simulink model "Simple_4Quad_payload_03"  (R2018b)
settings: Solver=VariableStepAuto  StartTime=0.0  StopTime=60  RelTol=1e-3
InitFcn:
  | Simple_4Quad_payload_03_const
values from neighbouring files (symbols this model uses):
  B = 1e0*eye(n)    [Simple_2Quad_payload_03_const.m]    (also in constant_CAMFC2_Quad_New_02_Payload_01.m = eye(n); test01.m = [eye(3) eye(3) eye(3) eye(3))
  BBT_inv = ((B'*B)^(-1))*B'    [Simple_2Quad_payload_03_const.m]    (also in Simple_4Quad_payload_04_const.m = ((BR'*BR)^(-1))*BR'; Simple_4Quad_payload_05_const.m = ((BR'*BR)^(-1))*BR'; Simple_4Quad_payload_06_const.m = ((BR'*BR)^(-1))*BR'; Simple_4Quad_payload_07_const.m = ((BR'*BR)^(-1))*BR')
  d1 = 0.25    [Colab_4Quad_model_01_const.m]    (also in Colab_4Quad_model_02_const.m = 0.5; Simple_4Quad_payload_01_const.m = 1; Simple_4Quad_payload_02_const.m = 1; Simple_4Quad_payload_03_const.m = 1)
  d2 = 0.25    [Colab_4Quad_model_01_const.m]    (also in Colab_4Quad_model_02_const.m = 0.5; Simple_4Quad_payload_01_const.m = 1; Simple_4Quad_payload_02_const.m = 1; Simple_4Quad_payload_03_const.m = 1)
  Des_rel_dist = 2    [Simple_4Quad_payload_01_const.m]    (also in Simple_4Quad_payload_02_const.m = 4; Simple_4Quad_payload_03_const.m = 4; Simple_4Quad_payload_04_const.m; Simple_4Quad_payload_05_const.m)
  gamma_0 = 1e-0*diag([1e-3;1e-0])    [Simple_2Quad_payload_03_const.m]    (also in Simple_4Quad_payload_04_const.m = 1e-0*diag([1e-6*ones(3,1);1e-0*ones(3,1)]); Simple_4Quad_payload_05_const.m = 1e-1*diag([1e-6*ones(3,1);1e-0*ones(3,1)]); Simple_4Quad_payload_06_const.m = 1e-0*diag([1e-6*ones(3,1);1e-0*ones(3,1)]); Simple_4Quad_payload_07_const.m = 1e-0*diag([1e-6*ones(3,1);1e-0*ones(3,1)]))
  gamma_1 = 1e+2*diag([1e-3;1e-0])    [Simple_2Quad_payload_03_const.m]    (also in Simple_4Quad_payload_04_const.m = 1e+2*diag([1e-6*ones(3,1);1e-0*ones(3,1)]); Simple_4Quad_payload_05_const.m = 1e+2*diag([1e-6*ones(3,1);1e-0*ones(3,1)]); Simple_4Quad_payload_06_const.m = 1e+3*diag([1e-6*ones(3,1);1e-0*ones(3,1)]); Simple_4Quad_payload_07_const.m = 1e+3*diag([1e-6*ones(3,1);1e-0*ones(3,1)]))
  ge = 9.81    [Simple_4Quad_payload_03_const.m]    (also in constant_CAMFC2_Quad_New_02_Payload_01.m)
  Ix = 0.166667    [Colab_4Quad_model_01_const.m]    (also in Colab_4Quad_model_02_const.m = 0.02; Simple_4Quad_payload_01_const.m = 1; Simple_4Quad_payload_02_const.m = 1; Simple_4Quad_payload_03_const.m = 1)
  Iy = 0.166667    [Colab_4Quad_model_01_const.m]    (also in Colab_4Quad_model_02_const.m = 0.02; Simple_4Quad_payload_01_const.m = 1; Simple_4Quad_payload_02_const.m = 1; Simple_4Quad_payload_03_const.m = 1)
  Iz = 0.166667    [Colab_4Quad_model_01_const.m]    (also in Colab_4Quad_model_02_const.m = 0.02; Simple_4Quad_payload_01_const.m = 1; Simple_4Quad_payload_02_const.m = 1; Simple_4Quad_payload_03_const.m = 1)
  Jq = diag([0.0291 0.0291 0.0552])    [Colab_4Quad_model_01_const.m]    (also in Colab_4Quad_model_02_const.m = diag([0.03 0.03 0.06]); Simple_4Quad_payload_03_const.m = 1.2416e-3 * diag([1 1 2]); Simple_4Quad_payload_04_const.m = 1 * diag([1 1 2]); Simple_4Quad_payload_05_const.m = 1 * diag([1 1 2]))
  k1 = 1    [Simple_2Quad_payload_03_const.m]    (also in Simple_4Quad_payload_04_const.m; Simple_4Quad_payload_05_const.m; Simple_4Quad_payload_06_const.m; Simple_4Quad_payload_07_const.m)
  k2 = 0.1    [Simple_2Quad_payload_03_const.m]    (also in Simple_4Quad_payload_04_const.m; Simple_4Quad_payload_05_const.m; Simple_4Quad_payload_06_const.m; Simple_4Quad_payload_07_const.m)
  Ka = 0.01    [Simple_4Quad_payload_03_const.m]    (also in constant_CAMFC2_Quad_New_02_Payload_01.m)
  Kd = 0.01    [Simple_4Quad_payload_03_const.m]    (also in constant_CAMFC2_Quad_New_02_Payload_01.m)
  Kf = 1.0e-5    (= 1e-05)    [Simple_4Quad_payload_03_const.m]    (also in constant_CAMFC2_Quad_New_02_Payload_01.m)
  ki1_N = 0    [Simple_4Quad_payload_02_const.m]    (also in Simple_4Quad_payload_03_const.m; Simple_4Quad_payload_04_const.m; Simple_4Quad_payload_05_const.m; Simple_4Quad_payload_06_const.m)
  ki1_S = 0    [Simple_4Quad_payload_02_const.m]    (also in Simple_4Quad_payload_03_const.m; Simple_4Quad_payload_04_const.m)
  ki2_N = 0    [Simple_4Quad_payload_02_const.m]    (also in Simple_4Quad_payload_03_const.m; Simple_4Quad_payload_04_const.m; Simple_4Quad_payload_05_const.m; Simple_4Quad_payload_06_const.m = 10)
  ki2_S = 0    [Simple_4Quad_payload_02_const.m]    (also in Simple_4Quad_payload_03_const.m; Simple_4Quad_payload_04_const.m)
  kp1_N = 10    [Simple_4Quad_payload_02_const.m]    (also in Simple_4Quad_payload_03_const.m; Simple_4Quad_payload_04_const.m; Simple_4Quad_payload_05_const.m = 1; Simple_4Quad_payload_06_const.m = 1)
  kp1_S = 10    [Simple_4Quad_payload_02_const.m]    (also in Simple_4Quad_payload_03_const.m; Simple_4Quad_payload_04_const.m)
  kp2_N = 100    [Simple_4Quad_payload_02_const.m]    (also in Simple_4Quad_payload_03_const.m; Simple_4Quad_payload_04_const.m; Simple_4Quad_payload_05_const.m = 1; Simple_4Quad_payload_06_const.m = 1)
  kp2_S = 100    [Simple_4Quad_payload_02_const.m]    (also in Simple_4Quad_payload_03_const.m; Simple_4Quad_payload_04_const.m)
  Kt = 0.0435 * Kf    (= 4.35e-07)    [Simple_4Quad_payload_03_const.m]    (also in constant_CAMFC2_Quad_New_02_Payload_01.m = 1e-07)
  l = 3.1819    [Colab_4Quad_model_01_const.m]    (also in Colab_4Quad_model_02_const.m = 3; Simple_2Quad_payload_04_const.m = 1; Simple_4Quad_payload_01_const.m = 1; Simple_4Quad_payload_02_const.m = 2)
  Lq = 0.45    [Simple_4Quad_payload_03_const.m]    (also in constant_CAMFC2_Quad_New_02_Payload_01.m = 0.2)
  m = 1.5    [Colab_4Quad_model_01_const.m]    (also in Colab_4Quad_model_02_const.m; Simple_2Quad_payload_04_const.m = 1; Simple_4Quad_payload_01_const.m = 1; Simple_4Quad_payload_02_const.m = 1)
  M = 1.0    (= 1)    [Colab_4Quad_model_01_const.m]    (also in Colab_4Quad_model_02_const.m; Simple_2Quad_payload_01_const.m; Simple_2Quad_payload_02_const.m; Simple_2Quad_payload_03_const.m)
  Md = 1*[1;1;1]    [Simple_2Quad_payload_04_const.m]    (also in Simple_4Quad_payload_01_const.m = 1*[1;1;1;1;1;1]; Simple_4Quad_payload_02_const.m = 1*[1;1;1;1;1;1]; Simple_4Quad_payload_03_const.m = 1*[1;1;1;1;1;1]; Simple_4Quad_payload_04_const.m = 1*[1;1;1;1;1;1])
  Mq = 2.95    [Simple_4Quad_payload_03_const.m]
  n = 2    [Simple_2Quad_payload_03_const.m]    (also in Simple_4Quad_payload_03_const.m = 6; Simple_4Quad_payload_04_const.m = 6; Simple_4Quad_payload_05_const.m = 6; Simple_4Quad_payload_06_const.m = 6)
  QR = 1e-0*eye(n)    [Simple_4Quad_payload_04_const.m]    (also in Simple_4Quad_payload_05_const.m = 1e-1*eye(n); Simple_4Quad_payload_06_const.m; Simple_4Quad_payload_07_const.m; Simple_4Quad_payload_08_const.m)
  R = 1e+0*eye(n)    [Simple_2Quad_payload_03_const.m]    (also in Simple_4Quad_payload_04_const.m = 1e+0*eye(m); Simple_4Quad_payload_05_const.m = 1e+0*eye(m); Simple_4Quad_payload_06_const.m; Simple_4Quad_payload_07_const.m)
  rho_0 = 1e-0    (= 1)    [Simple_2Quad_payload_03_const.m]    (also in Simple_4Quad_payload_04_const.m; Simple_4Quad_payload_05_const.m = 0.1; Simple_4Quad_payload_06_const.m; Simple_4Quad_payload_07_const.m)
  rho_1 = 1e-0    (= 1)    [Simple_2Quad_payload_03_const.m]    (also in Simple_4Quad_payload_04_const.m; Simple_4Quad_payload_05_const.m; Simple_4Quad_payload_06_const.m; Simple_4Quad_payload_07_const.m)
undefined symbols (not defined in the file or in its folder): mq
libraries: simulink x16
(part 1 of 3)
settings Model: Creator=ali  LastModifiedBy=ali

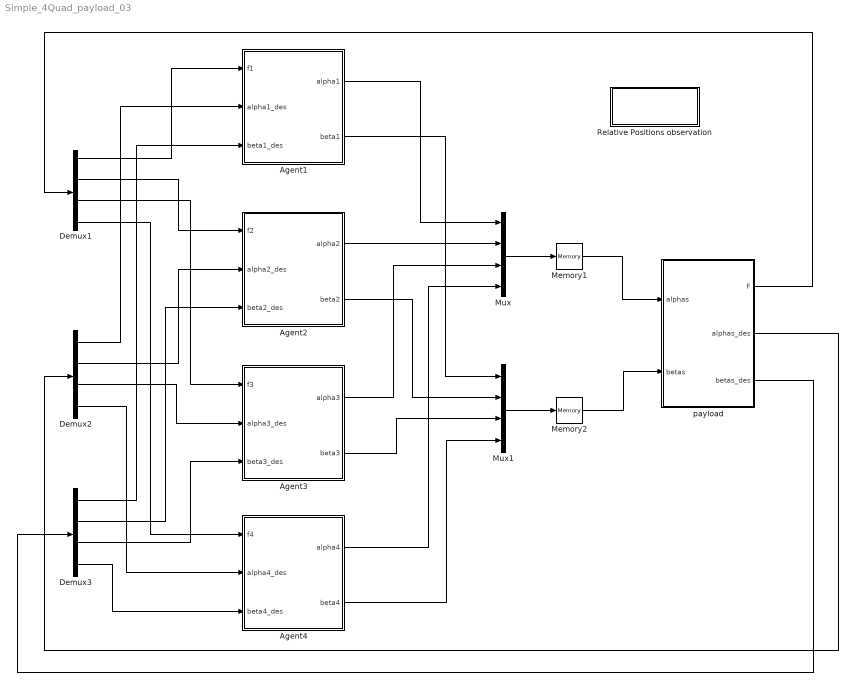
== system Simple_4Quad_payload_03 ==
  "Agent1 " : Subsystem
  Agent2 : Subsystem
  Agent3 : Subsystem
  Agent4 : Subsystem
  Demux1 : Demux
  Demux2 : Demux
  Demux3 : Demux
  Memory1 : Memory  InitialCondition=zeros(4,1)
  Memory2 : Memory  InitialCondition=zeros(4,1)
  Mux : Mux
  Mux1 : Mux
  Relative Positions observation : Subsystem
  payload : Subsystem
  wires:
  payload/1(F) -> Demux1/1
  payload/2(alphas_des) -> Demux2/1
  payload/3(betas_des) -> Demux3/1
  Demux1/1 -> "Agent1 "/1(f1)
  Demux1/2 -> Agent2/1(f2)
  Demux1/3 -> Agent3/1(f3)
  Demux1/4 -> Agent4/1(f4)
  Demux2/1 -> "Agent1 "/2(alpha1_des)
  Demux2/2 -> Agent2/2(alpha2_des)
  Demux2/3 -> Agent3/2(alpha3_des)
  Demux3/1 -> "Agent1 "/3(beta1_des)
  Demux3/2 -> Agent2/3(beta2_des)
  Demux3/3 -> Agent3/3(beta3_des)
  Demux2/4 -> Agent4/2(alpha4_des)
  Demux3/4 -> Agent4/3(beta4_des)
  "Agent1 "/1(alpha1) -> Mux/1
  Agent2/1(alpha2) -> Mux/2
  Agent3/1(alpha3) -> Mux/3
  Agent4/1(alpha4) -> Mux/4
  "Agent1 "/2(beta1) -> Mux1/1
  Agent2/2(beta2) -> Mux1/2
  Agent3/2(beta3) -> Mux1/3
  Agent4/2(beta4) -> Mux1/4
  Mux/1 -> Memory1/1
  Mux1/1 -> Memory2/1
  Memory2/1 -> payload/2(betas)
  Memory1/1 -> payload/1(alphas)

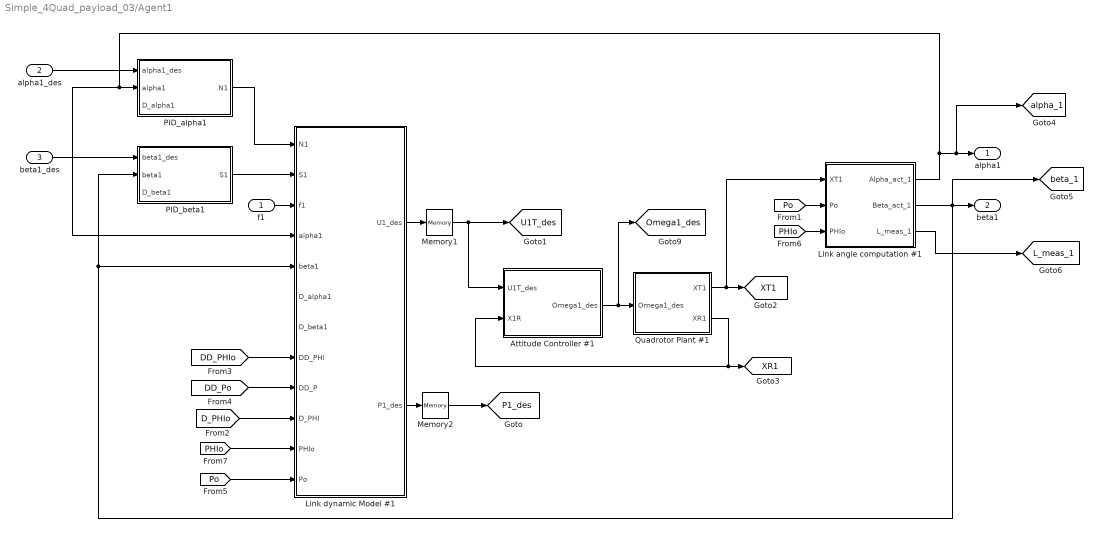
== system Simple_4Quad_payload_03/Agent1  ==
  f1 : Inport
  alpha1_des : Inport  Port=2
  beta1_des : Inport  Port=3
  Attitude Controller #1 : Subsystem
  Link angle computation #1 : MATLAB Function  TreatAsAtomicUnit=on
  Link dynamic Model #1 : MATLAB Function  TreatAsAtomicUnit=on
  Memory1 : Memory  InitialCondition=zeros(3,1)
  Memory2 : Memory  InitialCondition=zeros(3,1)
  PID_alpha1 : Subsystem
  PID_beta1 : Subsystem
  Quadrotor Plant #1 : Subsystem
  alpha1 : Outport
  beta1 : Outport  Port=2
  tag scope: L_meas_1=global, Omega1_des=global, P1_des=global, U1T_des=global, XR1=global, XT1=global, alpha_1=global, beta_1=global
  wires:
  PID_alpha1/1(N1) -> Link dynamic Model #1/1(N1)
  PID_beta1/1(S1) -> Link dynamic Model #1/2(S1)
  f1/1 -> Link dynamic Model #1/3(f1)
  Memory2/1 -> [P1_des]
  Memory1/1 -> Attitude Controller #1/1(U1T_des), [U1T_des]
  beta1_des/1 -> PID_beta1/1(beta1_des)
  [PHIo] -> Link dynamic Model #1/11(PHIo)
  [DD_Po] -> Link dynamic Model #1/9(DD_P)
  [D_PHIo] -> Link dynamic Model #1/10(D_PHI)
  [Po] -> Link dynamic Model #1/12(Po)
  [DD_PHIo] -> Link dynamic Model #1/8(DD_PHI)
  Link dynamic Model #1/1(U1_des) -> Memory1/1
  alpha1_des/1 -> PID_alpha1/1(alpha1_des)
  Link dynamic Model #1/2(P1_des) -> Memory2/1
  Quadrotor Plant #1/2(XR1) -> Attitude Controller #1/2(X1R), [XR1]
  Attitude Controller #1/1(Omega1_des) -> Quadrotor Plant #1/1(Omega1_des), [Omega1_des]
  Quadrotor Plant #1/1(XT1) -> Link angle computation #1/1(XT1), [XT1]
  Link angle computation #1/2(Beta_act_1) -> [beta_1], PID_beta1/2(beta1), Link dynamic Model #1/5(beta1), beta1/1
  Link angle computation #1/1(Alpha_act_1) -> Link dynamic Model #1/4(alpha1), PID_alpha1/2(alpha1), [alpha_1], alpha1/1
  [Po] -> Link angle computation #1/2(Po)
  [PHIo] -> Link angle computation #1/3(PHIo)
  Link angle computation #1/3(L_meas_1) -> [L_meas_1]

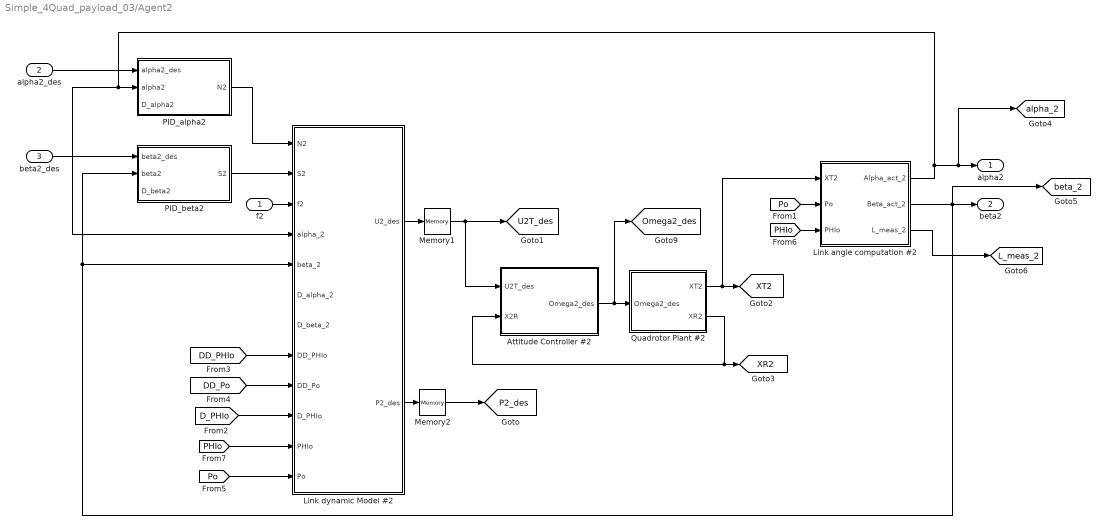
== system Simple_4Quad_payload_03/Agent2 ==
  f2 : Inport
  alpha2_des : Inport  Port=2
  beta2_des : Inport  Port=3
  Attitude Controller #2 : Subsystem
  Link angle computation #2 : MATLAB Function  TreatAsAtomicUnit=on
  Link dynamic Model #2 : MATLAB Function  TreatAsAtomicUnit=on
  Memory1 : Memory  InitialCondition=zeros(3,1)
  Memory2 : Memory  InitialCondition=zeros(3,1)
  PID_alpha2 : Subsystem
  PID_beta2 : Subsystem
  Quadrotor Plant #2 : Subsystem
  alpha2 : Outport
  beta2 : Outport  Port=2
  tag scope: L_meas_2=global, Omega2_des=global, P2_des=global, U2T_des=global, XR2=global, XT2=global, alpha_2=global, beta_2=global
  wires:
  PID_alpha2/1(N2) -> Link dynamic Model #2/1(N2)
  PID_beta2/1(S2) -> Link dynamic Model #2/2(S2)
  f2/1 -> Link dynamic Model #2/3(f2)
  Memory2/1 -> [P2_des]
  Memory1/1 -> Attitude Controller #2/1(U2T_des), [U2T_des]
  beta2_des/1 -> PID_beta2/1(beta2_des)
  [PHIo] -> Link dynamic Model #2/11(PHIo)
  [DD_Po] -> Link dynamic Model #2/9(DD_Po)
  [D_PHIo] -> Link dynamic Model #2/10(D_PHIo)
  [Po] -> Link dynamic Model #2/12(Po)
  [DD_PHIo] -> Link dynamic Model #2/8(DD_PHIo)
  Link dynamic Model #2/1(U2_des) -> Memory1/1
  alpha2_des/1 -> PID_alpha2/1(alpha2_des)
  Link dynamic Model #2/2(P2_des) -> Memory2/1
  Quadrotor Plant #2/2(XR2) -> Attitude Controller #2/2(X2R), [XR2]
  Attitude Controller #2/1(Omega2_des) -> Quadrotor Plant #2/1(Omega2_des), [Omega2_des]
  Quadrotor Plant #2/1(XT2) -> Link angle computation #2/1(XT2), [XT2]
  Link angle computation #2/2(Beta_act_2) -> [beta_2], PID_beta2/2(beta2), Link dynamic Model #2/5(beta_2), beta2/1
  Link angle computation #2/1(Alpha_act_2) -> Link dynamic Model #2/4(alpha_2), PID_alpha2/2(alpha2), [alpha_2], alpha2/1
  [Po] -> Link angle computation #2/2(Po)
  [PHIo] -> Link angle computation #2/3(PHIo)
  Link angle computation #2/3(L_meas_2) -> [L_meas_2]

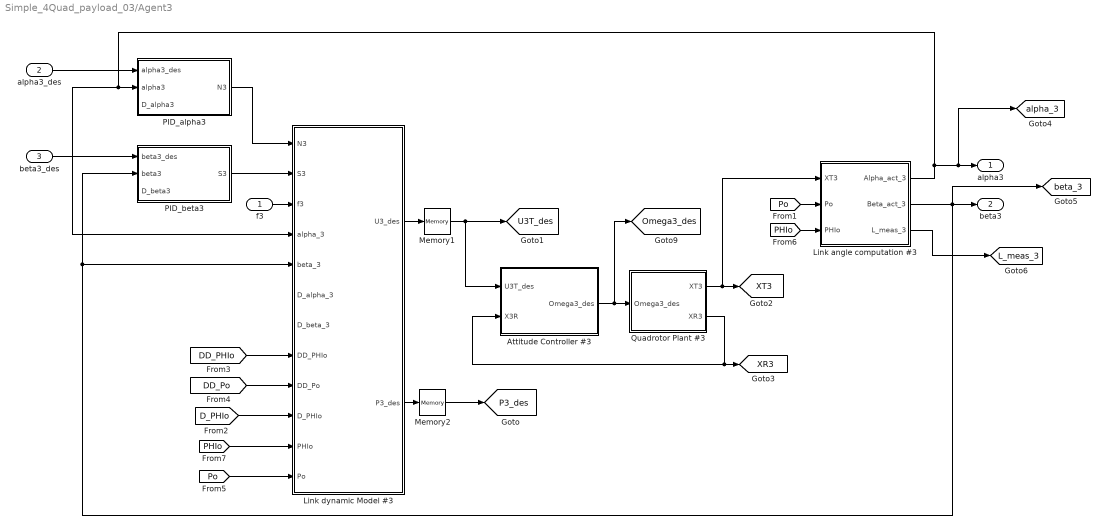
== system Simple_4Quad_payload_03/Agent3 ==
  f3 : Inport
  alpha3_des : Inport  Port=2
  beta3_des : Inport  Port=3
  Attitude Controller #3 : Subsystem
  Link angle computation #3 : MATLAB Function  TreatAsAtomicUnit=on
  Link dynamic Model #3 : MATLAB Function  TreatAsAtomicUnit=on
  Memory1 : Memory  InitialCondition=zeros(3,1)
  Memory2 : Memory  InitialCondition=zeros(3,1)
  PID_alpha3 : Subsystem
  PID_beta3 : Subsystem
  Quadrotor Plant #3 : Subsystem
  alpha3 : Outport
  beta3 : Outport  Port=2
  tag scope: L_meas_3=global, Omega3_des=global, P3_des=global, U3T_des=global, XR3=global, XT3=global, alpha_3=global, beta_3=global
  wires:
  Link angle computation #3/3(L_meas_3) -> [L_meas_3]
  [PHIo] -> Link angle computation #3/3(PHIo)
  [Po] -> Link angle computation #3/2(Po)
  Link angle computation #3/1(Alpha_act_3) -> alpha3/1, [alpha_3], PID_alpha3/2(alpha3), Link dynamic Model #3/4(alpha_3)
  Link angle computation #3/2(Beta_act_3) -> beta3/1, Link dynamic Model #3/5(beta_3), PID_beta3/2(beta3), [beta_3]
  Quadrotor Plant #3/1(XT3) -> [XT3], Link angle computation #3/1(XT3)
  Attitude Controller #3/1(Omega3_des) -> [Omega3_des], Quadrotor Plant #3/1(Omega3_des)
  Quadrotor Plant #3/2(XR3) -> [XR3], Attitude Controller #3/2(X3R)
  Link dynamic Model #3/2(P3_des) -> Memory2/1
  alpha3_des/1 -> PID_alpha3/1(alpha3_des)
  Link dynamic Model #3/1(U3_des) -> Memory1/1
  [DD_PHIo] -> Link dynamic Model #3/8(DD_PHIo)
  [Po] -> Link dynamic Model #3/12(Po)
  [D_PHIo] -> Link dynamic Model #3/10(D_PHIo)
  [DD_Po] -> Link dynamic Model #3/9(DD_Po)
  [PHIo] -> Link dynamic Model #3/11(PHIo)
  beta3_des/1 -> PID_beta3/1(beta3_des)
  Memory1/1 -> [U3T_des], Attitude Controller #3/1(U3T_des)
  Memory2/1 -> [P3_des]
  f3/1 -> Link dynamic Model #3/3(f3)
  PID_beta3/1(S3) -> Link dynamic Model #3/2(S3)
  PID_alpha3/1(N3) -> Link dynamic Model #3/1(N3)

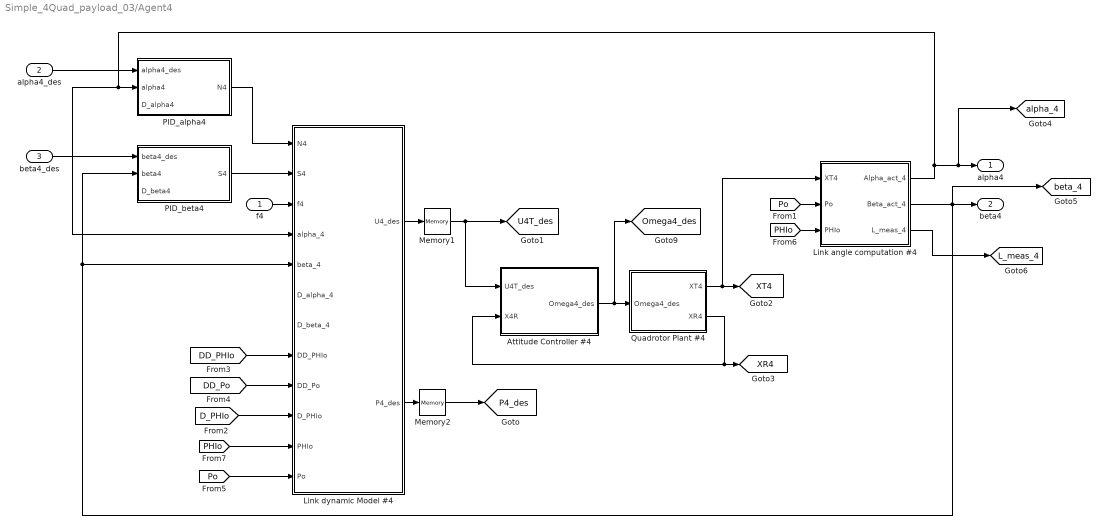
== system Simple_4Quad_payload_03/Agent4 ==
  f4 : Inport
  alpha4_des : Inport  Port=2
  beta4_des : Inport  Port=3
  Attitude Controller #4 : Subsystem
  Link angle computation #4 : MATLAB Function  TreatAsAtomicUnit=on
  Link dynamic Model #4 : MATLAB Function  TreatAsAtomicUnit=on
  Memory1 : Memory  InitialCondition=zeros(3,1)
  Memory2 : Memory  InitialCondition=zeros(3,1)
  PID_alpha4 : Subsystem
  PID_beta4 : Subsystem
  Quadrotor Plant #4 : Subsystem
  alpha4 : Outport
  beta4 : Outport  Port=2
  tag scope: L_meas_4=global, Omega4_des=global, P4_des=global, U4T_des=global, XR4=global, XT4=global, alpha_4=global, beta_4=global
  wires:
  PID_alpha4/1(N4) -> Link dynamic Model #4/1(N4)
  PID_beta4/1(S4) -> Link dynamic Model #4/2(S4)
  f4/1 -> Link dynamic Model #4/3(f4)
  Memory2/1 -> [P4_des]
  Memory1/1 -> Attitude Controller #4/1(U4T_des), [U4T_des]
  beta4_des/1 -> PID_beta4/1(beta4_des)
  [PHIo] -> Link dynamic Model #4/11(PHIo)
  [DD_Po] -> Link dynamic Model #4/9(DD_Po)
  [D_PHIo] -> Link dynamic Model #4/10(D_PHIo)
  [Po] -> Link dynamic Model #4/12(Po)
  [DD_PHIo] -> Link dynamic Model #4/8(DD_PHIo)
  Link dynamic Model #4/1(U4_des) -> Memory1/1
  alpha4_des/1 -> PID_alpha4/1(alpha4_des)
  Link dynamic Model #4/2(P4_des) -> Memory2/1
  Quadrotor Plant #4/2(XR4) -> Attitude Controller #4/2(X4R), [XR4]
  Attitude Controller #4/1(Omega4_des) -> Quadrotor Plant #4/1(Omega4_des), [Omega4_des]
  Quadrotor Plant #4/1(XT4) -> Link angle computation #4/1(XT4), [XT4]
  Link angle computation #4/2(Beta_act_4) -> [beta_4], PID_beta4/2(beta4), Link dynamic Model #4/5(beta_4), beta4/1
  Link angle computation #4/1(Alpha_act_4) -> Link dynamic Model #4/4(alpha_4), PID_alpha4/2(alpha4), [alpha_4], alpha4/1
  [Po] -> Link angle computation #4/2(Po)
  [PHIo] -> Link angle computation #4/3(PHIo)
  Link angle computation #4/3(L_meas_4) -> [L_meas_4]

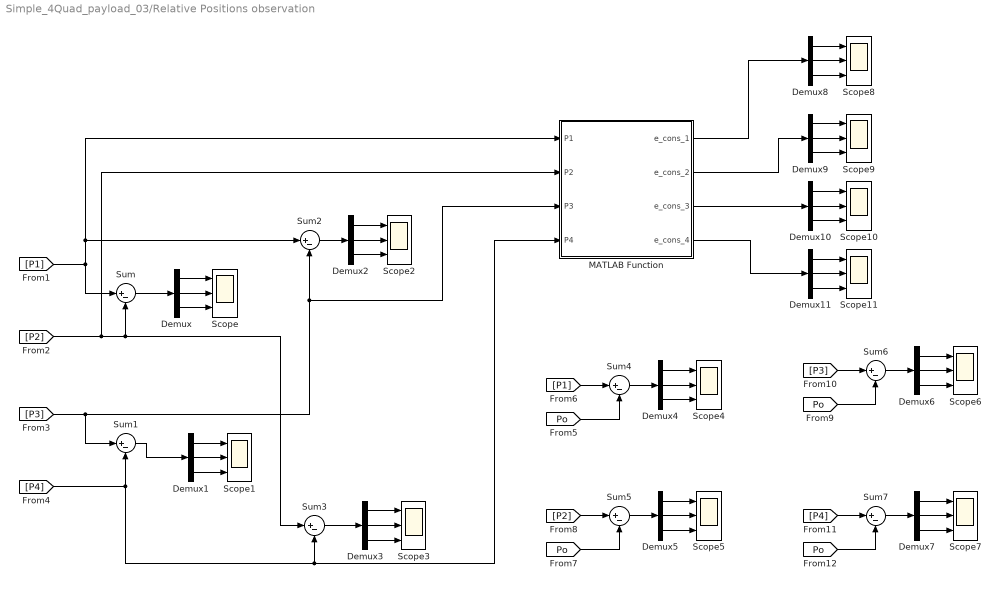
== system Simple_4Quad_payload_03/Relative Positions observation ==
  Demux{,1..11} (12 alike) : Demux  Outputs=3
  MATLAB Function : MATLAB Function  TreatAsAtomicUnit=on
  Scope{,1..11} (12 alike) : Scope  NumInputPorts=3
  Sum{,1..7} (8 alike) : Sum  Inputs=|+-
  wires:
  Demux/3 -> Scope/3
  Demux/1 -> Scope/1
  Demux/2 -> Scope/2
  Sum/1 -> Demux/1
  Sum1/1 -> Demux1/1
  Demux1/2 -> Scope1/2
  Demux1/1 -> Scope1/1
  Demux1/3 -> Scope1/3
  Sum2/1 -> Demux2/1
  [P3] -> MATLAB Function/3(P3), Sum2/2, Sum1/1
  [P1] -> Sum/1, MATLAB Function/1(P1), Sum2/1
  Demux2/2 -> Scope2/2
  Demux2/1 -> Scope2/1
  Demux2/3 -> Scope2/3
  Demux3/3 -> Scope3/3
  Demux3/1 -> Scope3/1
  Demux3/2 -> Scope3/2
  [P2] -> MATLAB Function/2(P2), Sum/2, Sum3/1
  [P4] -> Sum3/2, MATLAB Function/4(P4), Sum1/2
  Sum3/1 -> Demux3/1
  Demux4/3 -> Scope4/3
  Demux4/1 -> Scope4/1
  Demux4/2 -> Scope4/2
  Sum4/1 -> Demux4/1
  Sum5/1 -> Demux5/1
  Demux5/2 -> Scope5/2
  Demux5/1 -> Scope5/1
  Demux5/3 -> Scope5/3
  Demux6/3 -> Scope6/3
  Demux6/1 -> Scope6/1
  Demux6/2 -> Scope6/2
  Sum6/1 -> Demux6/1
  Sum7/1 -> Demux7/1
  Demux7/2 -> Scope7/2
  Demux7/1 -> Scope7/1
  Demux7/3 -> Scope7/3
  [Po] -> Sum4/2
  [P1] -> Sum4/1
  [P2] -> Sum5/1
  [Po] -> Sum5/2
  [P3] -> Sum6/1
  [Po] -> Sum6/2
  [P4] -> Sum7/1
  [Po] -> Sum7/2
  Demux8/2 -> Scope8/2
  Demux8/1 -> Scope8/1
  Demux8/3 -> Scope8/3
  MATLAB Function/1(e_cons_1) -> Demux8/1
  Demux9/3 -> Scope9/3
  Demux9/1 -> Scope9/1
  Demux9/2 -> Scope9/2
  MATLAB Function/2(e_cons_2) -> Demux9/1
  Demux10/2 -> Scope10/2
  Demux10/1 -> Scope10/1
  Demux10/3 -> Scope10/3
  MATLAB Function/3(e_cons_3) -> Demux10/1
  Demux11/3 -> Scope11/3
  Demux11/1 -> Scope11/1
  Demux11/2 -> Scope11/2
  MATLAB Function/4(e_cons_4) -> Demux11/1

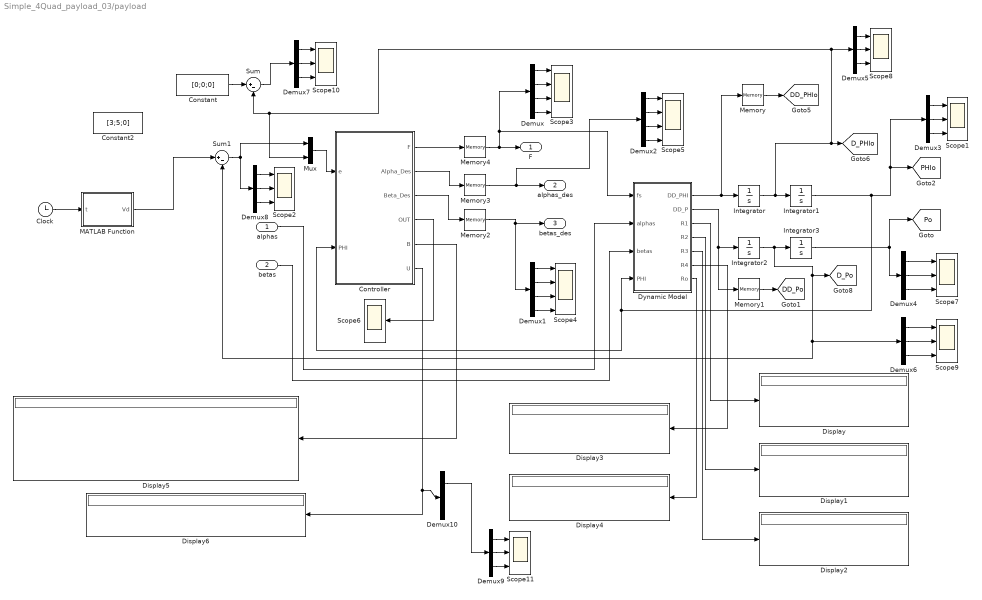
== system Simple_4Quad_payload_03/payload ==
  alphas : Inport
  betas : Inport  Port=2
  Clock : Clock
  Constant : Constant  Value=[0;0;0]
  Constant2 : Constant  Value=[3;5;0]
  Controller : MATLAB Function  TreatAsAtomicUnit=on
  Demux : Demux
  Demux1 : Demux
  Demux10 : Demux  Outputs=2
  Demux2 : Demux
  Demux{3..9} (7 alike) : Demux  Outputs=3
  Display{,1..6} (7 alike) : Display
  Dynamic Model : MATLAB Function  TreatAsAtomicUnit=on
  Integrator : Integrator  InitialCondition=zeros(3,1)
  Integrator1 : Integrator  InitialCondition=zeros(3,1)
  Integrator2 : Integrator  InitialCondition=zeros(3,1)
  Integrator3 : Integrator  InitialCondition=[0;0;0]
  MATLAB Function : MATLAB Function  TreatAsAtomicUnit=on
  Memory : Memory  InitialCondition=zeros(3,1)
  Memory1 : Memory  InitialCondition=zeros(3,1)
  Memory2 : Memory  InitialCondition=[0;pi;pi/2;-pi/2]
  Memory3 : Memory  InitialCondition=pi/2*ones(4,1)
  Memory4 : Memory  InitialCondition=zeros(4,1)
  Mux : Mux  Inputs=2
  Scope{1..2,7..11} (7 alike) : Scope  NumInputPorts=3
  Scope3 : Scope  NumInputPorts=4
  Scope4 : Scope  NumInputPorts=4
  Scope5 : Scope  NumInputPorts=4
  Scope6 : Scope
  Sum : Sum  Inputs=|+-
  Sum1 : Sum  Inputs=|+-
  F : Outport
  alphas_des : Outport  Port=2
  betas_des : Outport  Port=3
  tag scope: DD_PHIo=global, DD_Po=global, D_PHIo=global, D_Po=global, PHIo=global, Po=global
  wires:
  Dynamic Model/1(DD_PHI) -> Integrator/1, Memory/1
  Integrator/1 -> Integrator1/1, [D_PHIo], Demux5/1, Mux/2, Sum/2
  Integrator1/1 -> Demux3/1, [PHIo], Controller/2(PHI), Dynamic Model/4(PHI)
  Integrator2/1 -> Integrator3/1, [D_Po], Sum1/2, Demux6/1
  Dynamic Model/2(DD_P) -> Memory1/1, Integrator2/1
  alphas/1 -> Dynamic Model/2(alphas)
  Integrator3/1 -> [Po], Demux4/1
  Constant/1 -> Sum/1
  MATLAB Function/1(Vd) -> Sum1/1
  Memory/1 -> [DD_PHIo]
  Controller/4(OUT) -> Scope6/1
  Mux/1 -> Controller/1(e)
  betas/1 -> Dynamic Model/3(betas)
  Controller/1(F) -> Memory4/1
  Controller/2(Alpha_Des) -> Memory3/1
  Demux/1 -> Scope3/1
  Demux/2 -> Scope3/2
  Demux/3 -> Scope3/3
  Demux/4 -> Scope3/4
  Demux1/4 -> Scope4/4
  Demux1/3 -> Scope4/3
  Demux1/2 -> Scope4/2
  Demux1/1 -> Scope4/1
  Controller/3(Beta_Des) -> Memory2/1
  Demux2/1 -> Scope5/1
  Demux2/2 -> Scope5/2
  Demux2/3 -> Scope5/3
  Demux2/4 -> Scope5/4
  Demux3/3 -> Scope1/3
  Demux3/2 -> Scope1/2
  Demux3/1 -> Scope1/1
  Demux4/1 -> Scope7/1
  Demux4/2 -> Scope7/2
  Demux4/3 -> Scope7/3
  Memory1/1 -> [DD_Po]
  Demux5/1 -> Scope8/1
  Demux5/2 -> Scope8/2
  Demux5/3 -> Scope8/3
  Demux6/3 -> Scope9/3
  Demux6/2 -> Scope9/2
  Demux6/1 -> Scope9/1
  Sum1/1 -> Demux8/1, Mux/1
  Demux7/3 -> Scope10/3
  Demux7/2 -> Scope10/2
  Demux7/1 -> Scope10/1
  Demux8/1 -> Scope2/1
  Demux8/2 -> Scope2/2
  Demux8/3 -> Scope2/3
  Sum/1 -> Demux7/1
  Memory2/1 -> betas_des/1, Demux1/1
  Memory3/1 -> alphas_des/1, Demux2/1
  Memory4/1 -> Demux/1, Dynamic Model/1(fs), F/1
  Dynamic Model/3(R1) -> Display/1
  Dynamic Model/4(R2) -> Display1/1
  Dynamic Model/5(R3) -> Display2/1
  Dynamic Model/6(R4) -> Display3/1
  Dynamic Model/7(Ro) -> Display4/1
  Controller/5(B) -> Display5/1
  Controller/6(U) -> Demux10/1, Display6/1
  Demux9/1 -> Scope11/1
  Demux9/2 -> Scope11/2
  Demux9/3 -> Scope11/3
  Demux10/1 -> Demux9/1
  Clock/1 -> MATLAB Function/1(t)

== system Simple_4Quad_payload_03/Agent1 /Attitude Controller #1 ==
  U1T_des : Inport
  X1R : Inport  Port=2
  Controller Interpreter #1 : MATLAB Function  TreatAsAtomicUnit=on
  Controller to Motors #1 : MATLAB Function  TreatAsAtomicUnit=on
  Rotational #1 : Subsystem
  Scope : Scope
  Omega1_des : Outport
  wires:
  Rotational #1/1(ur1) -> Controller to Motors #1/2(uR1)
  U1T_des/1 -> Controller Interpreter #1/1(ut_1)
  X1R/1 -> Rotational #1/2(X)
  Controller to Motors #1/1(u_final_1) -> Omega1_des/1
  Controller Interpreter #1/1(uT_1) -> Controller to Motors #1/1(uT1)
  Controller Interpreter #1/2(PHI_d_1) -> Rotational #1/1(x_rd), Scope/1

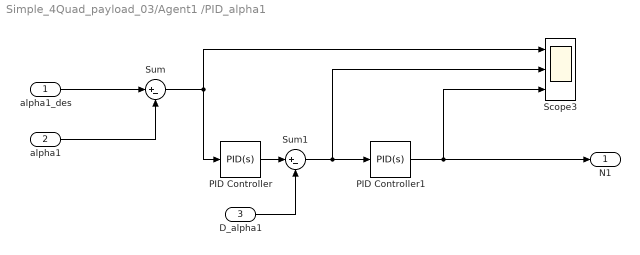
== system Simple_4Quad_payload_03/Agent1 /PID_alpha1 ==
  alpha1_des : Inport
  alpha1 : Inport  Port=2
  D_alpha1 : Inport  Port=3
  PID Controller : simulink/Continuous/PID Controller  Controller=PID  Form=Parallel  TimeDomain=Continuous-time  SampleTime=-1  IntegratorMethod=Forward Euler  FilterMethod=Forward Euler  ControllerParametersSource=internal  P=kp1_N  I=ki1_N  D=0  UseFilter=on  N=100  TunerSelectOption=Transfer Function Based (PID Tuner App)  InitialConditionSource=internal  InitialConditionForIntegrator=0  InitialConditionForFilter=0  DifferentiatorICPrevScaledInput=0  ExternalReset=none  TrackingMode=off  Kt=1  LimitOutput=off  UpperSaturationLimit=inf  LowerSaturationLimit=-inf  LinearizeAsGain=on  AntiWindupMode=none  Kb=1  POutMin=[]  POutMax=[]  IOutMin=[]  IOutMax=[]  DOutMin=[]  DOutMax=[]  NOutMin=[]  NOutMax=[]  SumOutMin=[]  SumOutMax=[]  SaturationOutMin=[]  SaturationOutMax=[]  PParamMin=[]  PParamMax=[]  IParamMin=[]  IParamMax=[]  DParamMin=[]  DParamMax=[]  NParamMin=[]  NParamMax=[]  KbParamMin=[]  KbParamMax=[]  KtParamMin=[]  KtParamMax=[]  KbOutMin=[]  KbOutMax=[]  KtOutMin=[]  KtOutMax=[]  IntegratorOutMin=[]  IntegratorOutMax=[]  FilterOutMin=[]  FilterOutMax=[]  SumI1OutMin=[]  SumI1OutMax=[]  SumI2OutMin=[]  SumI2OutMax=[]  SumI3OutMin=[]  SumI3OutMax=[]  SumI4OutMin=[]  SumI4OutMax=[]  SumDOutMin=[]  SumDOutMax=[]  DifferentiatorOutMin=[]  DifferentiatorOutMax=[]  FilterDiffOutCoefMin=[]  FilterDiffOutCoefMax=[]  ReciprocalOutMin=[]  ReciprocalOutMax=[]  SumDenOutMin=[]  SumDenOutMax=[]  SumNumOutMin=[]  SumNumOutMax=[]  DivideOutMin=[]  DivideOutMax=[]  IntegratorContinuousStateAttributes=''  IntegratorStateMustResolveToSignalObject=off  IntegratorRTWStateStorageClass=Auto  FilterContinuousStateAttributes=''  FilterStateMustResolveToSignalObject=off  FilterRTWStateStorageClass=Auto  ParallelPVariant=InternalParameters  IdealPVariant=Disabled  IVariant=InternalParameters  DVariant=InternalParameters  IntegratorVariant=Continuous  SatVariant=Disabled  AWVariant=Passthrough  PCopyVariant=Disabled  TRVariant=Disabled  FdbkBlocksVariant=Forward  IdealPFdbkVariant=Disabled  SatFdbkVariant=Disabled  DerivativeFilterVariant=ContFilter  NVariant=InternalParameters  NCopyVariant=Disabled  FilterICVariant=InternalICsFilter  IntegratorICVariant=InternalICs  ExternalResetVariant=Disabled  TRSumVariant=Passthrough  SumFdbkVariant=Disabled  SumVariant=Sum_PID
  PID Controller1 : simulink/Continuous/PID Controller  Controller=PID  Form=Parallel  TimeDomain=Continuous-time  SampleTime=-1  IntegratorMethod=Forward Euler  FilterMethod=Forward Euler  ControllerParametersSource=internal  P=kp2_N  I=ki2_N  D=0  UseFilter=on  N=100  TunerSelectOption=Transfer Function Based (PID Tuner App)  InitialConditionSource=internal  InitialConditionForIntegrator=0  InitialConditionForFilter=0  DifferentiatorICPrevScaledInput=0  ExternalReset=none  TrackingMode=off  Kt=1  LimitOutput=off  UpperSaturationLimit=inf  LowerSaturationLimit=-inf  LinearizeAsGain=on  AntiWindupMode=none  Kb=1  POutMin=[]  POutMax=[]  IOutMin=[]  IOutMax=[]  DOutMin=[]  DOutMax=[]  NOutMin=[]  NOutMax=[]  SumOutMin=[]  SumOutMax=[]  SaturationOutMin=[]  SaturationOutMax=[]  PParamMin=[]  PParamMax=[]  IParamMin=[]  IParamMax=[]  DParamMin=[]  DParamMax=[]  NParamMin=[]  NParamMax=[]  KbParamMin=[]  KbParamMax=[]  KtParamMin=[]  KtParamMax=[]  KbOutMin=[]  KbOutMax=[]  KtOutMin=[]  KtOutMax=[]  IntegratorOutMin=[]  IntegratorOutMax=[]  FilterOutMin=[]  FilterOutMax=[]  SumI1OutMin=[]  SumI1OutMax=[]  SumI2OutMin=[]  SumI2OutMax=[]  SumI3OutMin=[]  SumI3OutMax=[]  SumI4OutMin=[]  SumI4OutMax=[]  SumDOutMin=[]  SumDOutMax=[]  DifferentiatorOutMin=[]  DifferentiatorOutMax=[]  FilterDiffOutCoefMin=[]  FilterDiffOutCoefMax=[]  ReciprocalOutMin=[]  ReciprocalOutMax=[]  SumDenOutMin=[]  SumDenOutMax=[]  SumNumOutMin=[]  SumNumOutMax=[]  DivideOutMin=[]  DivideOutMax=[]  IntegratorContinuousStateAttributes=''  IntegratorStateMustResolveToSignalObject=off  IntegratorRTWStateStorageClass=Auto  FilterContinuousStateAttributes=''  FilterStateMustResolveToSignalObject=off  FilterRTWStateStorageClass=Auto  ParallelPVariant=InternalParameters  IdealPVariant=Disabled  IVariant=InternalParameters  DVariant=InternalParameters  IntegratorVariant=Continuous  SatVariant=Disabled  AWVariant=Passthrough  PCopyVariant=Disabled  TRVariant=Disabled  FdbkBlocksVariant=Forward  IdealPFdbkVariant=Disabled  SatFdbkVariant=Disabled  DerivativeFilterVariant=ContFilter  NVariant=InternalParameters  NCopyVariant=Disabled  FilterICVariant=InternalICsFilter  IntegratorICVariant=InternalICs  ExternalResetVariant=Disabled  TRSumVariant=Passthrough  SumFdbkVariant=Disabled  SumVariant=Sum_PID
  Scope3 : Scope  NumInputPorts=3
  Sum : Sum  Inputs=|+-
  Sum1 : Sum  Inputs=|+-
  N1 : Outport
  wires:
  D_alpha1/1 -> Sum1/2
  alpha1/1 -> Sum/2
  alpha1_des/1 -> Sum/1
  Sum1/1 -> Scope3/2, PID Controller1/1
  Sum/1 -> PID Controller/1, Scope3/1
  PID Controller1/1 -> Scope3/3, N1/1
  PID Controller/1 -> Sum1/1

== system Simple_4Quad_payload_03/Agent1 /PID_beta1 ==
  beta1_des : Inport
  beta1 : Inport  Port=2
  D_beta1 : Inport  Port=3
  PID Controller : simulink/Continuous/PID Controller  Controller=PID  Form=Parallel  TimeDomain=Continuous-time  SampleTime=-1  IntegratorMethod=Forward Euler  FilterMethod=Forward Euler  ControllerParametersSource=internal  P=kp1_S  I=ki1_S  D=0  UseFilter=on  N=100  TunerSelectOption=Transfer Function Based (PID Tuner App)  InitialConditionSource=internal  InitialConditionForIntegrator=0  InitialConditionForFilter=0  DifferentiatorICPrevScaledInput=0  ExternalReset=none  TrackingMode=off  Kt=1  LimitOutput=off  UpperSaturationLimit=inf  LowerSaturationLimit=-inf  LinearizeAsGain=on  AntiWindupMode=none  Kb=1  POutMin=[]  POutMax=[]  IOutMin=[]  IOutMax=[]  DOutMin=[]  DOutMax=[]  NOutMin=[]  NOutMax=[]  SumOutMin=[]  SumOutMax=[]  SaturationOutMin=[]  SaturationOutMax=[]  PParamMin=[]  PParamMax=[]  IParamMin=[]  IParamMax=[]  DParamMin=[]  DParamMax=[]  NParamMin=[]  NParamMax=[]  KbParamMin=[]  KbParamMax=[]  KtParamMin=[]  KtParamMax=[]  KbOutMin=[]  KbOutMax=[]  KtOutMin=[]  KtOutMax=[]  IntegratorOutMin=[]  IntegratorOutMax=[]  FilterOutMin=[]  FilterOutMax=[]  SumI1OutMin=[]  SumI1OutMax=[]  SumI2OutMin=[]  SumI2OutMax=[]  SumI3OutMin=[]  SumI3OutMax=[]  SumI4OutMin=[]  SumI4OutMax=[]  SumDOutMin=[]  SumDOutMax=[]  DifferentiatorOutMin=[]  DifferentiatorOutMax=[]  FilterDiffOutCoefMin=[]  FilterDiffOutCoefMax=[]  ReciprocalOutMin=[]  ReciprocalOutMax=[]  SumDenOutMin=[]  SumDenOutMax=[]  SumNumOutMin=[]  SumNumOutMax=[]  DivideOutMin=[]  DivideOutMax=[]  IntegratorContinuousStateAttributes=''  IntegratorStateMustResolveToSignalObject=off  IntegratorRTWStateStorageClass=Auto  FilterContinuousStateAttributes=''  FilterStateMustResolveToSignalObject=off  FilterRTWStateStorageClass=Auto  ParallelPVariant=InternalParameters  IdealPVariant=Disabled  IVariant=InternalParameters  DVariant=InternalParameters  IntegratorVariant=Continuous  SatVariant=Disabled  AWVariant=Passthrough  PCopyVariant=Disabled  TRVariant=Disabled  FdbkBlocksVariant=Forward  IdealPFdbkVariant=Disabled  SatFdbkVariant=Disabled  DerivativeFilterVariant=ContFilter  NVariant=InternalParameters  NCopyVariant=Disabled  FilterICVariant=InternalICsFilter  IntegratorICVariant=InternalICs  ExternalResetVariant=Disabled  TRSumVariant=Passthrough  SumFdbkVariant=Disabled  SumVariant=Sum_PID
  PID Controller1 : simulink/Continuous/PID Controller  Controller=PID  Form=Parallel  TimeDomain=Continuous-time  SampleTime=-1  IntegratorMethod=Forward Euler  FilterMethod=Forward Euler  ControllerParametersSource=internal  P=kp2_S  I=ki2_S  D=0  UseFilter=on  N=100  TunerSelectOption=Transfer Function Based (PID Tuner App)  InitialConditionSource=internal  InitialConditionForIntegrator=0  InitialConditionForFilter=0  DifferentiatorICPrevScaledInput=0  ExternalReset=none  TrackingMode=off  Kt=1  LimitOutput=off  UpperSaturationLimit=inf  LowerSaturationLimit=-inf  LinearizeAsGain=on  AntiWindupMode=none  Kb=1  POutMin=[]  POutMax=[]  IOutMin=[]  IOutMax=[]  DOutMin=[]  DOutMax=[]  NOutMin=[]  NOutMax=[]  SumOutMin=[]  SumOutMax=[]  SaturationOutMin=[]  SaturationOutMax=[]  PParamMin=[]  PParamMax=[]  IParamMin=[]  IParamMax=[]  DParamMin=[]  DParamMax=[]  NParamMin=[]  NParamMax=[]  KbParamMin=[]  KbParamMax=[]  KtParamMin=[]  KtParamMax=[]  KbOutMin=[]  KbOutMax=[]  KtOutMin=[]  KtOutMax=[]  IntegratorOutMin=[]  IntegratorOutMax=[]  FilterOutMin=[]  FilterOutMax=[]  SumI1OutMin=[]  SumI1OutMax=[]  SumI2OutMin=[]  SumI2OutMax=[]  SumI3OutMin=[]  SumI3OutMax=[]  SumI4OutMin=[]  SumI4OutMax=[]  SumDOutMin=[]  SumDOutMax=[]  DifferentiatorOutMin=[]  DifferentiatorOutMax=[]  FilterDiffOutCoefMin=[]  FilterDiffOutCoefMax=[]  ReciprocalOutMin=[]  ReciprocalOutMax=[]  SumDenOutMin=[]  SumDenOutMax=[]  SumNumOutMin=[]  SumNumOutMax=[]  DivideOutMin=[]  DivideOutMax=[]  IntegratorContinuousStateAttributes=''  IntegratorStateMustResolveToSignalObject=off  IntegratorRTWStateStorageClass=Auto  FilterContinuousStateAttributes=''  FilterStateMustResolveToSignalObject=off  FilterRTWStateStorageClass=Auto  ParallelPVariant=InternalParameters  IdealPVariant=Disabled  IVariant=InternalParameters  DVariant=InternalParameters  IntegratorVariant=Continuous  SatVariant=Disabled  AWVariant=Passthrough  PCopyVariant=Disabled  TRVariant=Disabled  FdbkBlocksVariant=Forward  IdealPFdbkVariant=Disabled  SatFdbkVariant=Disabled  DerivativeFilterVariant=ContFilter  NVariant=InternalParameters  NCopyVariant=Disabled  FilterICVariant=InternalICsFilter  IntegratorICVariant=InternalICs  ExternalResetVariant=Disabled  TRSumVariant=Passthrough  SumFdbkVariant=Disabled  SumVariant=Sum_PID
  Scope3 : Scope  NumInputPorts=3
  Sum : Sum  Inputs=|+-
  Sum1 : Sum  Inputs=|+-
  S1 : Outport
  wires:
  D_beta1/1 -> Sum1/2
  PID Controller/1 -> Sum1/1
  PID Controller1/1 -> S1/1, Scope3/3
  Sum/1 -> Scope3/1, PID Controller/1
  Sum1/1 -> PID Controller1/1, Scope3/2
  beta1_des/1 -> Sum/1
  beta1/1 -> Sum/2

== system Simple_4Quad_payload_03/Agent1 /Quadrotor Plant #1 ==
  Omega1_des : Inport
  Clock : Clock
  Integrator : Integrator  InitialCondition=zeros(n,1)
  Integrator1 : Integrator  InitialCondition=zeros(n,1)
  MATLAB Function : MATLAB Function  TreatAsAtomicUnit=on
  XT1 : Outport
  XR1 : Outport  Port=2
  wires:
  Clock/1 -> MATLAB Function/4(t)
  MATLAB Function/1(D_XT1) -> Integrator/1
  Integrator/1 -> XT1/1, MATLAB Function/1(XT1)
  Integrator1/1 -> XR1/1, MATLAB Function/2(XR1)
  MATLAB Function/2(D_XR1) -> Integrator1/1
  Omega1_des/1 -> MATLAB Function/3(Omega1_des)

== system Simple_4Quad_payload_03/Agent2/Attitude Controller #2 ==
  U2T_des : Inport
  X2R : Inport  Port=2
  Controller Interpreter #2 : MATLAB Function  TreatAsAtomicUnit=on
  Controller to Motors #2 : MATLAB Function  TreatAsAtomicUnit=on
  Rotational #2 : Subsystem
  Scope : Scope
  Omega2_des : Outport
  wires:
  Rotational #2/1(ur) -> Controller to Motors #2/2(uR2)
  U2T_des/1 -> Controller Interpreter #2/1(ut_2)
  X2R/1 -> Rotational #2/2(X)
  Controller to Motors #2/1(u_final_2) -> Omega2_des/1
  Controller Interpreter #2/1(uT_2) -> Controller to Motors #2/1(uT2)
  Controller Interpreter #2/2(PHI_d_2) -> Rotational #2/1(x_rd), Scope/1

== system Simple_4Quad_payload_03/Agent2/PID_alpha2 ==
  alpha2_des : Inport
  alpha2 : Inport  Port=2
  D_alpha2 : Inport  Port=3
  PID Controller : simulink/Continuous/PID Controller  Controller=PID  Form=Parallel  TimeDomain=Continuous-time  SampleTime=-1  IntegratorMethod=Forward Euler  FilterMethod=Forward Euler  ControllerParametersSource=internal  P=kp1_N  I=ki1_N  D=0  UseFilter=on  N=100  TunerSelectOption=Transfer Function Based (PID Tuner App)  InitialConditionSource=internal  InitialConditionForIntegrator=0  InitialConditionForFilter=0  DifferentiatorICPrevScaledInput=0  ExternalReset=none  TrackingMode=off  Kt=1  LimitOutput=off  UpperSaturationLimit=inf  LowerSaturationLimit=-inf  LinearizeAsGain=on  AntiWindupMode=none  Kb=1  POutMin=[]  POutMax=[]  IOutMin=[]  IOutMax=[]  DOutMin=[]  DOutMax=[]  NOutMin=[]  NOutMax=[]  SumOutMin=[]  SumOutMax=[]  SaturationOutMin=[]  SaturationOutMax=[]  PParamMin=[]  PParamMax=[]  IParamMin=[]  IParamMax=[]  DParamMin=[]  DParamMax=[]  NParamMin=[]  NParamMax=[]  KbParamMin=[]  KbParamMax=[]  KtParamMin=[]  KtParamMax=[]  KbOutMin=[]  KbOutMax=[]  KtOutMin=[]  KtOutMax=[]  IntegratorOutMin=[]  IntegratorOutMax=[]  FilterOutMin=[]  FilterOutMax=[]  SumI1OutMin=[]  SumI1OutMax=[]  SumI2OutMin=[]  SumI2OutMax=[]  SumI3OutMin=[]  SumI3OutMax=[]  SumI4OutMin=[]  SumI4OutMax=[]  SumDOutMin=[]  SumDOutMax=[]  DifferentiatorOutMin=[]  DifferentiatorOutMax=[]  FilterDiffOutCoefMin=[]  FilterDiffOutCoefMax=[]  ReciprocalOutMin=[]  ReciprocalOutMax=[]  SumDenOutMin=[]  SumDenOutMax=[]  SumNumOutMin=[]  SumNumOutMax=[]  DivideOutMin=[]  DivideOutMax=[]  IntegratorContinuousStateAttributes=''  IntegratorStateMustResolveToSignalObject=off  IntegratorRTWStateStorageClass=Auto  FilterContinuousStateAttributes=''  FilterStateMustResolveToSignalObject=off  FilterRTWStateStorageClass=Auto  ParallelPVariant=InternalParameters  IdealPVariant=Disabled  IVariant=InternalParameters  DVariant=InternalParameters  IntegratorVariant=Continuous  SatVariant=Disabled  AWVariant=Passthrough  PCopyVariant=Disabled  TRVariant=Disabled  FdbkBlocksVariant=Forward  IdealPFdbkVariant=Disabled  SatFdbkVariant=Disabled  DerivativeFilterVariant=ContFilter  NVariant=InternalParameters  NCopyVariant=Disabled  FilterICVariant=InternalICsFilter  IntegratorICVariant=InternalICs  ExternalResetVariant=Disabled  TRSumVariant=Passthrough  SumFdbkVariant=Disabled  SumVariant=Sum_PID
  PID Controller1 : simulink/Continuous/PID Controller  Controller=PID  Form=Parallel  TimeDomain=Continuous-time  SampleTime=-1  IntegratorMethod=Forward Euler  FilterMethod=Forward Euler  ControllerParametersSource=internal  P=kp2_N  I=ki2_N  D=0  UseFilter=on  N=100  TunerSelectOption=Transfer Function Based (PID Tuner App)  InitialConditionSource=internal  InitialConditionForIntegrator=0  InitialConditionForFilter=0  DifferentiatorICPrevScaledInput=0  ExternalReset=none  TrackingMode=off  Kt=1  LimitOutput=off  UpperSaturationLimit=inf  LowerSaturationLimit=-inf  LinearizeAsGain=on  AntiWindupMode=none  Kb=1  POutMin=[]  POutMax=[]  IOutMin=[]  IOutMax=[]  DOutMin=[]  DOutMax=[]  NOutMin=[]  NOutMax=[]  SumOutMin=[]  SumOutMax=[]  SaturationOutMin=[]  SaturationOutMax=[]  PParamMin=[]  PParamMax=[]  IParamMin=[]  IParamMax=[]  DParamMin=[]  DParamMax=[]  NParamMin=[]  NParamMax=[]  KbParamMin=[]  KbParamMax=[]  KtParamMin=[]  KtParamMax=[]  KbOutMin=[]  KbOutMax=[]  KtOutMin=[]  KtOutMax=[]  IntegratorOutMin=[]  IntegratorOutMax=[]  FilterOutMin=[]  FilterOutMax=[]  SumI1OutMin=[]  SumI1OutMax=[]  SumI2OutMin=[]  SumI2OutMax=[]  SumI3OutMin=[]  SumI3OutMax=[]  SumI4OutMin=[]  SumI4OutMax=[]  SumDOutMin=[]  SumDOutMax=[]  DifferentiatorOutMin=[]  DifferentiatorOutMax=[]  FilterDiffOutCoefMin=[]  FilterDiffOutCoefMax=[]  ReciprocalOutMin=[]  ReciprocalOutMax=[]  SumDenOutMin=[]  SumDenOutMax=[]  SumNumOutMin=[]  SumNumOutMax=[]  DivideOutMin=[]  DivideOutMax=[]  IntegratorContinuousStateAttributes=''  IntegratorStateMustResolveToSignalObject=off  IntegratorRTWStateStorageClass=Auto  FilterContinuousStateAttributes=''  FilterStateMustResolveToSignalObject=off  FilterRTWStateStorageClass=Auto  ParallelPVariant=InternalParameters  IdealPVariant=Disabled  IVariant=InternalParameters  DVariant=InternalParameters  IntegratorVariant=Continuous  SatVariant=Disabled  AWVariant=Passthrough  PCopyVariant=Disabled  TRVariant=Disabled  FdbkBlocksVariant=Forward  IdealPFdbkVariant=Disabled  SatFdbkVariant=Disabled  DerivativeFilterVariant=ContFilter  NVariant=InternalParameters  NCopyVariant=Disabled  FilterICVariant=InternalICsFilter  IntegratorICVariant=InternalICs  ExternalResetVariant=Disabled  TRSumVariant=Passthrough  SumFdbkVariant=Disabled  SumVariant=Sum_PID
  Sum : Sum  Inputs=|+-
  Sum1 : Sum  Inputs=|+-
  N2 : Outport
  wires:
  D_alpha2/1 -> Sum1/2
  alpha2/1 -> Sum/2
  alpha2_des/1 -> Sum/1
  Sum1/1 -> PID Controller1/1
  Sum/1 -> PID Controller/1
  PID Controller1/1 -> N2/1
  PID Controller/1 -> Sum1/1

== system Simple_4Quad_payload_03/Agent2/PID_beta2 ==
  beta2_des : Inport
  beta2 : Inport  Port=2
  D_beta2 : Inport  Port=3
  PID Controller : simulink/Continuous/PID Controller  Controller=PID  Form=Parallel  TimeDomain=Continuous-time  SampleTime=-1  IntegratorMethod=Forward Euler  FilterMethod=Forward Euler  ControllerParametersSource=internal  P=kp1_S  I=ki1_S  D=0  UseFilter=on  N=100  TunerSelectOption=Transfer Function Based (PID Tuner App)  InitialConditionSource=internal  InitialConditionForIntegrator=0  InitialConditionForFilter=0  DifferentiatorICPrevScaledInput=0  ExternalReset=none  TrackingMode=off  Kt=1  LimitOutput=off  UpperSaturationLimit=inf  LowerSaturationLimit=-inf  LinearizeAsGain=on  AntiWindupMode=none  Kb=1  POutMin=[]  POutMax=[]  IOutMin=[]  IOutMax=[]  DOutMin=[]  DOutMax=[]  NOutMin=[]  NOutMax=[]  SumOutMin=[]  SumOutMax=[]  SaturationOutMin=[]  SaturationOutMax=[]  PParamMin=[]  PParamMax=[]  IParamMin=[]  IParamMax=[]  DParamMin=[]  DParamMax=[]  NParamMin=[]  NParamMax=[]  KbParamMin=[]  KbParamMax=[]  KtParamMin=[]  KtParamMax=[]  KbOutMin=[]  KbOutMax=[]  KtOutMin=[]  KtOutMax=[]  IntegratorOutMin=[]  IntegratorOutMax=[]  FilterOutMin=[]  FilterOutMax=[]  SumI1OutMin=[]  SumI1OutMax=[]  SumI2OutMin=[]  SumI2OutMax=[]  SumI3OutMin=[]  SumI3OutMax=[]  SumI4OutMin=[]  SumI4OutMax=[]  SumDOutMin=[]  SumDOutMax=[]  DifferentiatorOutMin=[]  DifferentiatorOutMax=[]  FilterDiffOutCoefMin=[]  FilterDiffOutCoefMax=[]  ReciprocalOutMin=[]  ReciprocalOutMax=[]  SumDenOutMin=[]  SumDenOutMax=[]  SumNumOutMin=[]  SumNumOutMax=[]  DivideOutMin=[]  DivideOutMax=[]  IntegratorContinuousStateAttributes=''  IntegratorStateMustResolveToSignalObject=off  IntegratorRTWStateStorageClass=Auto  FilterContinuousStateAttributes=''  FilterStateMustResolveToSignalObject=off  FilterRTWStateStorageClass=Auto  ParallelPVariant=InternalParameters  IdealPVariant=Disabled  IVariant=InternalParameters  DVariant=InternalParameters  IntegratorVariant=Continuous  SatVariant=Disabled  AWVariant=Passthrough  PCopyVariant=Disabled  TRVariant=Disabled  FdbkBlocksVariant=Forward  IdealPFdbkVariant=Disabled  SatFdbkVariant=Disabled  DerivativeFilterVariant=ContFilter  NVariant=InternalParameters  NCopyVariant=Disabled  FilterICVariant=InternalICsFilter  IntegratorICVariant=InternalICs  ExternalResetVariant=Disabled  TRSumVariant=Passthrough  SumFdbkVariant=Disabled  SumVariant=Sum_PID
  PID Controller1 : simulink/Continuous/PID Controller  Controller=PID  Form=Parallel  TimeDomain=Continuous-time  SampleTime=-1  IntegratorMethod=Forward Euler  FilterMethod=Forward Euler  ControllerParametersSource=internal  P=kp2_S  I=ki2_S  D=0  UseFilter=on  N=100  TunerSelectOption=Transfer Function Based (PID Tuner App)  InitialConditionSource=internal  InitialConditionForIntegrator=0  InitialConditionForFilter=0  DifferentiatorICPrevScaledInput=0  ExternalReset=none  TrackingMode=off  Kt=1  LimitOutput=off  UpperSaturationLimit=inf  LowerSaturationLimit=-inf  LinearizeAsGain=on  AntiWindupMode=none  Kb=1  POutMin=[]  POutMax=[]  IOutMin=[]  IOutMax=[]  DOutMin=[]  DOutMax=[]  NOutMin=[]  NOutMax=[]  SumOutMin=[]  SumOutMax=[]  SaturationOutMin=[]  SaturationOutMax=[]  PParamMin=[]  PParamMax=[]  IParamMin=[]  IParamMax=[]  DParamMin=[]  DParamMax=[]  NParamMin=[]  NParamMax=[]  KbParamMin=[]  KbParamMax=[]  KtParamMin=[]  KtParamMax=[]  KbOutMin=[]  KbOutMax=[]  KtOutMin=[]  KtOutMax=[]  IntegratorOutMin=[]  IntegratorOutMax=[]  FilterOutMin=[]  FilterOutMax=[]  SumI1OutMin=[]  SumI1OutMax=[]  SumI2OutMin=[]  SumI2OutMax=[]  SumI3OutMin=[]  SumI3OutMax=[]  SumI4OutMin=[]  SumI4OutMax=[]  SumDOutMin=[]  SumDOutMax=[]  DifferentiatorOutMin=[]  DifferentiatorOutMax=[]  FilterDiffOutCoefMin=[]  FilterDiffOutCoefMax=[]  ReciprocalOutMin=[]  ReciprocalOutMax=[]  SumDenOutMin=[]  SumDenOutMax=[]  SumNumOutMin=[]  SumNumOutMax=[]  DivideOutMin=[]  DivideOutMax=[]  IntegratorContinuousStateAttributes=''  IntegratorStateMustResolveToSignalObject=off  IntegratorRTWStateStorageClass=Auto  FilterContinuousStateAttributes=''  FilterStateMustResolveToSignalObject=off  FilterRTWStateStorageClass=Auto  ParallelPVariant=InternalParameters  IdealPVariant=Disabled  IVariant=InternalParameters  DVariant=InternalParameters  IntegratorVariant=Continuous  SatVariant=Disabled  AWVariant=Passthrough  PCopyVariant=Disabled  TRVariant=Disabled  FdbkBlocksVariant=Forward  IdealPFdbkVariant=Disabled  SatFdbkVariant=Disabled  DerivativeFilterVariant=ContFilter  NVariant=InternalParameters  NCopyVariant=Disabled  FilterICVariant=InternalICsFilter  IntegratorICVariant=InternalICs  ExternalResetVariant=Disabled  TRSumVariant=Passthrough  SumFdbkVariant=Disabled  SumVariant=Sum_PID
  Sum : Sum  Inputs=|+-
  Sum1 : Sum  Inputs=|+-
  S2 : Outport
  wires:
  D_beta2/1 -> Sum1/2
  PID Controller/1 -> Sum1/1
  PID Controller1/1 -> S2/1
  Sum/1 -> PID Controller/1
  Sum1/1 -> PID Controller1/1
  beta2_des/1 -> Sum/1
  beta2/1 -> Sum/2

== system Simple_4Quad_payload_03/Agent2/Quadrotor Plant #2 ==
  Omega2_des : Inport
  Clock : Clock
  Integrator : Integrator  InitialCondition=zeros(n,1)
  Integrator1 : Integrator  InitialCondition=zeros(n,1)
  MATLAB Function : MATLAB Function  TreatAsAtomicUnit=on
  XT2 : Outport
  XR2 : Outport  Port=2
  wires:
  Clock/1 -> MATLAB Function/4(t)
  MATLAB Function/1(D_XT2) -> Integrator/1
  Integrator/1 -> XT2/1, MATLAB Function/1(XT2)
  Integrator1/1 -> XR2/1, MATLAB Function/2(XR2)
  MATLAB Function/2(D_XR2) -> Integrator1/1
  Omega2_des/1 -> MATLAB Function/3(Omega2_des)

== system Simple_4Quad_payload_03/Agent3/Attitude Controller #3 ==
  U3T_des : Inport
  X3R : Inport  Port=2
  Controller Interpreter #3 : MATLAB Function  TreatAsAtomicUnit=on
  Controller to Motors #3 : MATLAB Function  TreatAsAtomicUnit=on
  Rotational #3 : Subsystem
  Scope : Scope
  Omega3_des : Outport
  wires:
  Controller Interpreter #3/2(PHI_d_3) -> Scope/1, Rotational #3/1(x_rd)
  Controller Interpreter #3/1(uT_3) -> Controller to Motors #3/1(uT3)
  Controller to Motors #3/1(u_final_3) -> Omega3_des/1
  X3R/1 -> Rotational #3/2(X)
  U3T_des/1 -> Controller Interpreter #3/1(ut_3)
  Rotational #3/1(ur) -> Controller to Motors #3/2(uR3)

== system Simple_4Quad_payload_03/Agent3/PID_alpha3 ==
  alpha3_des : Inport
  alpha3 : Inport  Port=2
  D_alpha3 : Inport  Port=3
  PID Controller : simulink/Continuous/PID Controller  Controller=PID  Form=Parallel  TimeDomain=Continuous-time  SampleTime=-1  IntegratorMethod=Forward Euler  FilterMethod=Forward Euler  ControllerParametersSource=internal  P=kp1_N  I=ki1_N  D=0  UseFilter=on  N=100  TunerSelectOption=Transfer Function Based (PID Tuner App)  InitialConditionSource=internal  InitialConditionForIntegrator=0  InitialConditionForFilter=0  DifferentiatorICPrevScaledInput=0  ExternalReset=none  TrackingMode=off  Kt=1  LimitOutput=off  UpperSaturationLimit=inf  LowerSaturationLimit=-inf  LinearizeAsGain=on  AntiWindupMode=none  Kb=1  POutMin=[]  POutMax=[]  IOutMin=[]  IOutMax=[]  DOutMin=[]  DOutMax=[]  NOutMin=[]  NOutMax=[]  SumOutMin=[]  SumOutMax=[]  SaturationOutMin=[]  SaturationOutMax=[]  PParamMin=[]  PParamMax=[]  IParamMin=[]  IParamMax=[]  DParamMin=[]  DParamMax=[]  NParamMin=[]  NParamMax=[]  KbParamMin=[]  KbParamMax=[]  KtParamMin=[]  KtParamMax=[]  KbOutMin=[]  KbOutMax=[]  KtOutMin=[]  KtOutMax=[]  IntegratorOutMin=[]  IntegratorOutMax=[]  FilterOutMin=[]  FilterOutMax=[]  SumI1OutMin=[]  SumI1OutMax=[]  SumI2OutMin=[]  SumI2OutMax=[]  SumI3OutMin=[]  SumI3OutMax=[]  SumI4OutMin=[]  SumI4OutMax=[]  SumDOutMin=[]  SumDOutMax=[]  DifferentiatorOutMin=[]  DifferentiatorOutMax=[]  FilterDiffOutCoefMin=[]  FilterDiffOutCoefMax=[]  ReciprocalOutMin=[]  ReciprocalOutMax=[]  SumDenOutMin=[]  SumDenOutMax=[]  SumNumOutMin=[]  SumNumOutMax=[]  DivideOutMin=[]  DivideOutMax=[]  IntegratorContinuousStateAttributes=''  IntegratorStateMustResolveToSignalObject=off  IntegratorRTWStateStorageClass=Auto  FilterContinuousStateAttributes=''  FilterStateMustResolveToSignalObject=off  FilterRTWStateStorageClass=Auto  ParallelPVariant=InternalParameters  IdealPVariant=Disabled  IVariant=InternalParameters  DVariant=InternalParameters  IntegratorVariant=Continuous  SatVariant=Disabled  AWVariant=Passthrough  PCopyVariant=Disabled  TRVariant=Disabled  FdbkBlocksVariant=Forward  IdealPFdbkVariant=Disabled  SatFdbkVariant=Disabled  DerivativeFilterVariant=ContFilter  NVariant=InternalParameters  NCopyVariant=Disabled  FilterICVariant=InternalICsFilter  IntegratorICVariant=InternalICs  ExternalResetVariant=Disabled  TRSumVariant=Passthrough  SumFdbkVariant=Disabled  SumVariant=Sum_PID
  PID Controller1 : simulink/Continuous/PID Controller  Controller=PID  Form=Parallel  TimeDomain=Continuous-time  SampleTime=-1  IntegratorMethod=Forward Euler  FilterMethod=Forward Euler  ControllerParametersSource=internal  P=kp2_N  I=ki2_N  D=0  UseFilter=on  N=100  TunerSelectOption=Transfer Function Based (PID Tuner App)  InitialConditionSource=internal  InitialConditionForIntegrator=0  InitialConditionForFilter=0  DifferentiatorICPrevScaledInput=0  ExternalReset=none  TrackingMode=off  Kt=1  LimitOutput=off  UpperSaturationLimit=inf  LowerSaturationLimit=-inf  LinearizeAsGain=on  AntiWindupMode=none  Kb=1  POutMin=[]  POutMax=[]  IOutMin=[]  IOutMax=[]  DOutMin=[]  DOutMax=[]  NOutMin=[]  NOutMax=[]  SumOutMin=[]  SumOutMax=[]  SaturationOutMin=[]  SaturationOutMax=[]  PParamMin=[]  PParamMax=[]  IParamMin=[]  IParamMax=[]  DParamMin=[]  DParamMax=[]  NParamMin=[]  NParamMax=[]  KbParamMin=[]  KbParamMax=[]  KtParamMin=[]  KtParamMax=[]  KbOutMin=[]  KbOutMax=[]  KtOutMin=[]  KtOutMax=[]  IntegratorOutMin=[]  IntegratorOutMax=[]  FilterOutMin=[]  FilterOutMax=[]  SumI1OutMin=[]  SumI1OutMax=[]  SumI2OutMin=[]  SumI2OutMax=[]  SumI3OutMin=[]  SumI3OutMax=[]  SumI4OutMin=[]  SumI4OutMax=[]  SumDOutMin=[]  SumDOutMax=[]  DifferentiatorOutMin=[]  DifferentiatorOutMax=[]  FilterDiffOutCoefMin=[]  FilterDiffOutCoefMax=[]  ReciprocalOutMin=[]  ReciprocalOutMax=[]  SumDenOutMin=[]  SumDenOutMax=[]  SumNumOutMin=[]  SumNumOutMax=[]  DivideOutMin=[]  DivideOutMax=[]  IntegratorContinuousStateAttributes=''  IntegratorStateMustResolveToSignalObject=off  IntegratorRTWStateStorageClass=Auto  FilterContinuousStateAttributes=''  FilterStateMustResolveToSignalObject=off  FilterRTWStateStorageClass=Auto  ParallelPVariant=InternalParameters  IdealPVariant=Disabled  IVariant=InternalParameters  DVariant=InternalParameters  IntegratorVariant=Continuous  SatVariant=Disabled  AWVariant=Passthrough  PCopyVariant=Disabled  TRVariant=Disabled  FdbkBlocksVariant=Forward  IdealPFdbkVariant=Disabled  SatFdbkVariant=Disabled  DerivativeFilterVariant=ContFilter  NVariant=InternalParameters  NCopyVariant=Disabled  FilterICVariant=InternalICsFilter  IntegratorICVariant=InternalICs  ExternalResetVariant=Disabled  TRSumVariant=Passthrough  SumFdbkVariant=Disabled  SumVariant=Sum_PID
  Sum : Sum  Inputs=|+-
  Sum1 : Sum  Inputs=|+-
  N3 : Outport
  wires:
  PID Controller/1 -> Sum1/1
  PID Controller1/1 -> N3/1
  Sum/1 -> PID Controller/1
  Sum1/1 -> PID Controller1/1
  alpha3_des/1 -> Sum/1
  alpha3/1 -> Sum/2
  D_alpha3/1 -> Sum1/2
